simulink model "Modelo_Amortiguacion"  (R2023b)
settings: Solver=ode45  StartTime=0  StopTime=10  FixedStep=1  RelTol=1e-3
values from neighbouring files (symbols this model uses):
  CI = {struct(x0=0.25, dx0=1), struct(Cc=30, mc=60, mr=12, Kc=20, Kr=700, Tp=randi([1, 5], 1), Tf=randi([3, 6], 1)), }    [sim_utils.m]
libraries: SignalEditorBlockLib x1
settings Model: Creator=alfre  LastModifiedBy=alfre

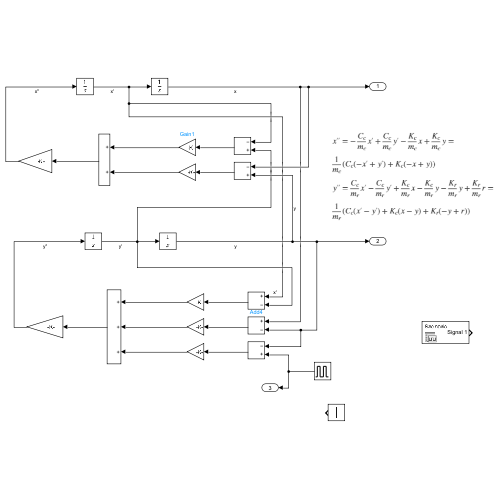
[thumbnail: Simulink's stored preview of the top-level diagram]
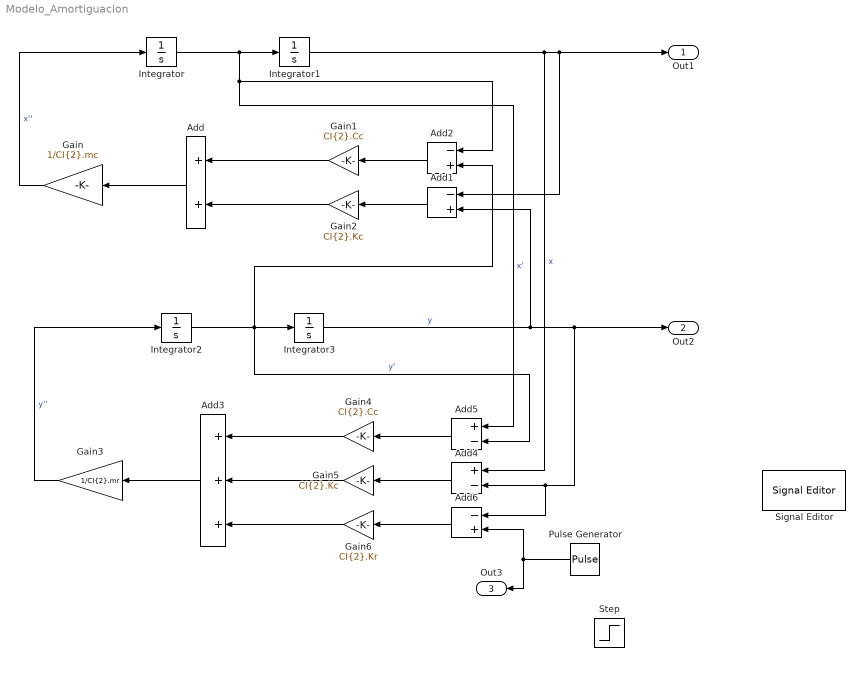
== system Modelo_Amortiguacion ==
  Add : Sum
  Add1 : Sum  Inputs=-+
  Add2 : Sum  Inputs=-+
  Add3 : Sum  Inputs=+++
  Add4 : Sum  Inputs=+-
  Add5 : Sum  Inputs=+-
  Add6 : Sum  Inputs=-+
  Gain : Gain  Gain=1/CI{2}.mc
  Gain1 : Gain  Gain=CI{2}.Cc
  Gain2 : Gain  Gain=CI{2}.Kc
  Gain3 : Gain  Gain=1/CI{2}.mr
  Gain4 : Gain  Gain=CI{2}.Cc
  Gain5 : Gain  Gain=CI{2}.Kc
  Gain6 : Gain  Gain=CI{2}.Kr
  Integrator{,1..3} (4 alike) : Integrator
  Pulse Generator : DiscretePulseGenerator  PulseType=Time based  Period=CI{2}.Tf  PulseWidth=CI{2}.Tp
  Signal Editor : SignalEditorBlockLib/Signal Editor  FileName=untitled.mat  ActiveScenario=Scenario  ActiveSignal=Signal 1  IsBus=off  OutputBusObjectStr=Bus: BusObject  SampleTime=0  Interpolate=off  ZeroCross=off  OutputAfterFinalValue=Setting to zero  Unit=inherit  PreserveSignalName=on  ApplySigPropsToAllScenarios=on  ApplySigPropsToAllSignals=off
  Step : Step  SampleTime=0
  Out1 : Outport
  Out2 : Outport  Port=2
  Out3 : Outport  Port=3
  wires:
  Integrator/1 -> Add5/1, Add2/1, Integrator1/1  "x'"
  Gain/1 -> Integrator/1  "x''"
  Integrator1/1 -> Add4/1, Out1/1, Add1/1  "x"
  Add/1 -> Gain/1
  Add2/1 -> Gain1/1
  Gain1/1 -> Add/1
  Gain2/1 -> Add/2
  Add1/1 -> Gain2/1
  Add5/1 -> Gain4/1
  Gain4/1 -> Add3/1
  Integrator3/1 -> Add1/2, Out2/1, Add4/2, Add6/1  "y"
  Add3/1 -> Gain3/1
  Add4/1 -> Gain5/1
  Integrator2/1 -> Integrator3/1, Add5/2, Add2/2  "y'"
  Gain5/1 -> Add3/2
  Gain3/1 -> Integrator2/1  "y''"
  Add6/1 -> Gain6/1
  Gain6/1 -> Add3/3
  Pulse Generator/1 -> Out3/1, Add6/2
